simulink model "fixed_references_test_model1"  (R2022b)
settings: Solver=VariableStepAuto  StartTime=0.0  StopTime=0.5  MaxStep=Tstep  RelTol=1e-3
InitFcn:
  | VDCrated=200;
  | Pbase=10e3;
undefined symbols (not defined in the file): I1_ref, I2_ref, I3_ref, V1_offset, V2_offset, V3_offset
libraries: simulink x1
settings Model: Creator=ajunyent  LastModifiedBy=IceSunYX

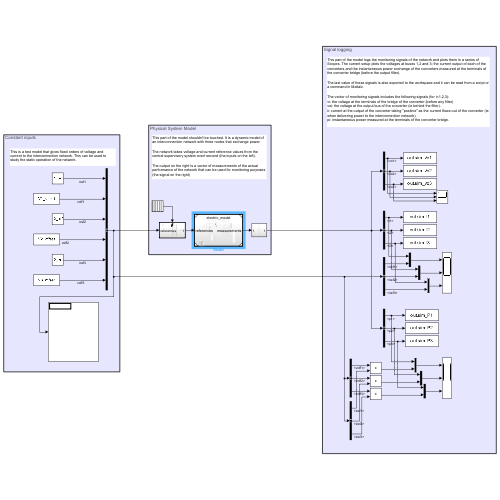
[thumbnail: Simulink's stored preview of the top-level diagram]
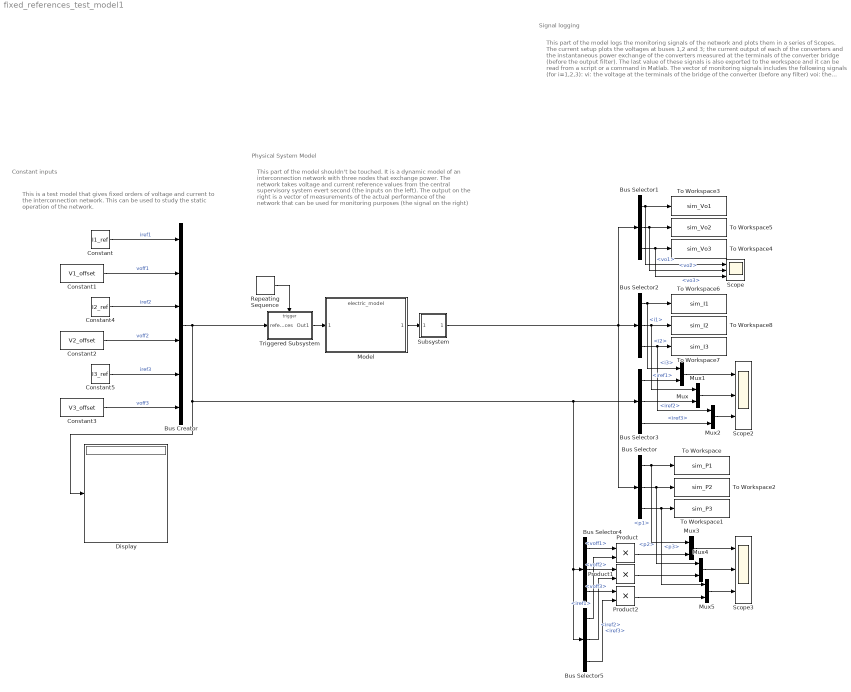
== system fixed_references_test_model1 ==
  note: This is a test model that gives fixed orders of voltage and current to the interconnection network. This can be used to study the static operation of the network.
  note: Constant inputs
  note: This part of the model shouldn't be touched. It is a dynamic model of an interconnection network with three nodes that exchange power.
      |
      | The network takes voltage and current reference values from the central supervisory system evert second (the inputs on the left).
      |
      | The output on the right is a vector of measurements of the actual performance of the network that can be used for monitoring purposes (the signal on the right)
  note: Physical System Model
  note: Signal logging
  note: This part of the model logs the monitoring signals of the network and plots them in a series of Scopes. The current setup plots the voltages at buses 1,2 and 3; the current output of each of the converters and the instantaneous power exchange of the converters measured at the terminals of the converter bridge (before the output filter).
      |
      | The last value of these signals is also exported to the workspace and it can be read from a script or a command in Matlab.
      |
      | The vector of monitoring signals includes the following signals (for i=1,2,3):
      | vi: the voltage at the terminals of the bridge of the converter (before any filter)
      | voi: the voltage at the output bus of the converter (ie behind the filter).
      | ii: current at the output of the converter taking "positive" as the current flows out of the converter (ie when delivering power to the interconnection network).
      | pi: instantaneous power measured at the terminals of the converter bridge.
  Bus Creator : BusCreator  Inputs=6
  Bus Selector : BusSelector  OutputSignals=p1,p2,p3
  Bus Selector1 : BusSelector  OutputSignals=vo1,vo2,vo3
  Bus Selector2 : BusSelector  OutputSignals=i1,i2,i3
  Bus Selector3 : BusSelector  OutputSignals=iref1,iref2,iref3
  Bus Selector4 : BusSelector  OutputSignals=voff1,voff2,voff3
  Bus Selector5 : BusSelector  OutputSignals=iref1,iref2,iref3
  Constant : Constant  Value=I1_ref
  Constant1 : Constant  Value=V1_offset
  Constant2 : Constant  Value=V2_offset
  Constant3 : Constant  Value=V3_offset
  Constant4 : Constant  Value=I2_ref
  Constant5 : Constant  Value=I3_ref
  Display : Display
  Model : ModelReference  ModelNameDialog=electric_model.slx  SimulationMode=Normal  ModelReferenceVersion=2.0
  Mux{,1..5} (6 alike) : Mux  Inputs=2
  Product : Product
  Product1 : Product
  Product2 : Product
  Repeating Sequence : simulink/Sources/Repeating Sequence  rep_seq_t=[0 0.005 0.006 0.5 0.501 1]  rep_seq_y=[0,0,1 1 0 0]
  Scope : Scope  NumInputPorts=3
  Scope2 : Scope  NumInputPorts=3
  Scope3 : Scope  NumInputPorts=3
  Subsystem : Subsystem
  To Workspace : ToWorkspace  VariableName=sim_P1  SampleTime=-1
      settings: MaxDataPoints=1
  To Workspace1 : ToWorkspace  VariableName=sim_P3  SampleTime=-1
      settings: MaxDataPoints=1
  To Workspace2 : ToWorkspace  VariableName=sim_P2  SampleTime=-1
      settings: MaxDataPoints=1
  To Workspace3 : ToWorkspace  VariableName=sim_Vo1  SampleTime=-1
      settings: MaxDataPoints=1
  To Workspace4 : ToWorkspace  VariableName=sim_Vo3  SampleTime=-1
      settings: MaxDataPoints=1
  To Workspace5 : ToWorkspace  VariableName=sim_Vo2  SampleTime=-1
      settings: MaxDataPoints=1
  To Workspace6 : ToWorkspace  VariableName=sim_I1  SampleTime=-1
      settings: MaxDataPoints=1
  To Workspace7 : ToWorkspace  VariableName=sim_I3  SampleTime=-1
      settings: MaxDataPoints=1
  To Workspace8 : ToWorkspace  VariableName=sim_I2  SampleTime=-1
      settings: MaxDataPoints=1
  Triggered Subsystem : Subsystem  TreatAsAtomicUnit=on
  wires:
  Constant1/1 -> Bus Creator/2  "voff1"
  Constant4/1 -> Bus Creator/3  "iref2"
  Constant5/1 -> Bus Creator/5  "iref3"
  Constant3/1 -> Bus Creator/6  "voff3"
  Model/1 -> Subsystem/1(In1)
  Triggered Subsystem/1(Out1) -> Model/1
  Constant/1 -> Bus Creator/1  "iref1"
  Repeating Sequence/1 -> Triggered Subsystem/Trigger
  Constant2/1 -> Bus Creator/4  "voff2"
  Bus Selector1/3 -> To Workspace4/1, Scope/3  "<vo3>"
  Bus Creator/1 -> Display/1, Bus Selector3/1, Bus Selector5/1, Bus Selector4/1, Triggered Subsystem/1(references)
  Bus Selector5/1 -> Product/2  "<iref1>"
  Product2/1 -> Mux5/2
  Bus Selector4/1 -> Product/1  "<voff1>"
  Mux1/1 -> Scope2/2
  Bus Selector1/2 -> To Workspace5/1, Scope/2  "<vo2>"
  Bus Selector3/3 -> Mux2/2  "<iref3>"
  Mux5/1 -> Scope3/3
  Product1/1 -> Mux4/2
  Bus Selector2/2 -> To Workspace8/1, Mux1/1  "<i2>"
  Bus Selector/3 -> Mux5/1, To Workspace1/1  "<p3>"
  Bus Selector2/3 -> Mux2/1, To Workspace7/1  "<i3>"
  Subsystem/1(Out1) -> Bus Selector/1, Bus Selector1/1, Bus Selector2/1
  Product/1 -> Mux3/2
  Mux/1 -> Scope2/1
  Mux2/1 -> Scope2/3
  Bus Selector/1 -> Mux3/1, To Workspace/1  "<p1>"
  Bus Selector/2 -> To Workspace2/1, Mux4/1  "<p2>"
  Bus Selector4/3 -> Product2/1  "<voff3>"
  Bus Selector1/1 -> To Workspace3/1, Scope/1  "<vo1>"
  Bus Selector5/2 -> Product1/2  "<iref2>"
  Bus Selector3/2 -> Mux1/2  "<iref2>"
  Bus Selector4/2 -> Product1/1  "<voff2>"
  Bus Selector3/1 -> Mux/2  "<iref1>"
  Bus Selector2/1 -> To Workspace6/1, Mux/1  "<i1>"
  Mux4/1 -> Scope3/2
  Mux3/1 -> Scope3/1
  Bus Selector5/3 -> Product2/2  "<iref3>"

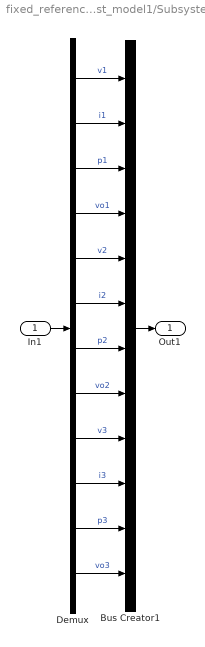
== system fixed_references_test_model1/Subsystem ==
  In1 : Inport
  Bus Creator1 : BusCreator  Inputs=12
  Demux : Demux  Outputs=12
  Out1 : Outport
  wires:
  Demux/2 -> Bus Creator1/2  "i1"
  Bus Creator1/1 -> Out1/1
  Demux/4 -> Bus Creator1/4  "vo1"
  Demux/1 -> Bus Creator1/1  "v1"
  Demux/11 -> Bus Creator1/11  "p3"
  Demux/5 -> Bus Creator1/5  "v2"
  In1/1 -> Demux/1
  Demux/10 -> Bus Creator1/10  "i3"
  Demux/8 -> Bus Creator1/8  "vo2"
  Demux/7 -> Bus Creator1/7  "p2"
  Demux/3 -> Bus Creator1/3  "p1"
  Demux/12 -> Bus Creator1/12  "vo3"
  Demux/9 -> Bus Creator1/9  "v3"
  Demux/6 -> Bus Creator1/6  "i2"

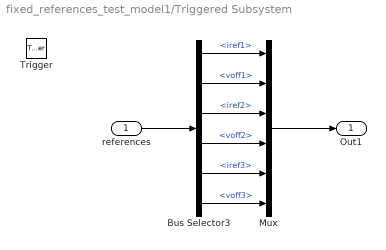
== system fixed_references_test_model1/Triggered Subsystem ==
  references : Inport
  Trigger : TriggerPort  VariantControl=(inherit)  InitialTriggerSignalState=zero
  Bus Selector3 : BusSelector  OutputSignals=iref1,voff1,iref2,voff2,iref3,voff3
  Mux : Mux  Inputs=6
  Out1 : Outport  InitialOutput=[0,VDCrated,0,VDCrated,0,VDCrated]
  wires:
  Bus Selector3/2 -> Mux/2  "<voff1>"
  Bus Selector3/4 -> Mux/4  "<voff2>"
  Bus Selector3/1 -> Mux/1  "<iref1>"
  Bus Selector3/5 -> Mux/5  "<iref3>"
  Bus Selector3/6 -> Mux/6  "<voff3>"
  Mux/1 -> Out1/1
  Bus Selector3/3 -> Mux/3  "<iref2>"
  references/1 -> Bus Selector3/1
